simulink model "software_assignment_2"  (R2025a)
settings: Solver=VariableStepAuto  StartTime=0.0  StopTime=10.0  RelTol=1e-3
settings Model: Creator=nikul  LastModifiedBy=nikul

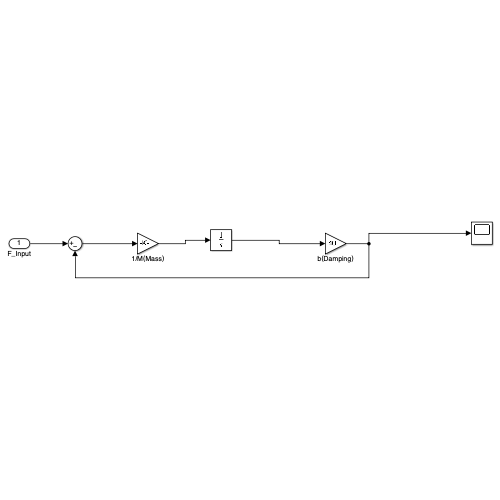
[thumbnail: Simulink's stored preview of the top-level diagram]
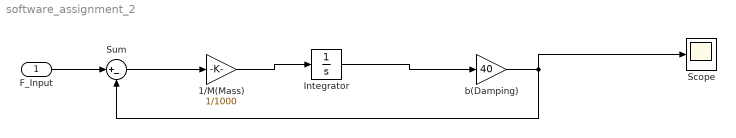
== system software_assignment_2 ==
  F_Input : Inport
  1/M(Mass) : Gain  Gain=1/1000
  Integrator : Integrator
  Scope : Scope
  Sum : Sum  Inputs=|+-
  b(Damping) : Gain  Gain=40
  wires:
  Integrator/1 -> b(Damping)/1
  b(Damping)/1 -> Scope/1, Sum/2
  Sum/1 -> 1/M(Mass)/1
  1/M(Mass)/1 -> Integrator/1
  F_Input/1 -> Sum/1
